simulink model "untitled1"  (R2024a)
settings: Solver=VariableStepAuto  StartTime=0.0  StopTime=10.0  RelTol=1e-3
undefined symbols (not defined in the file or in its folder): Discrete, pInitialization, Time
libraries: ctrlSharedLib x11, simulink x6
settings Model: Creator=DELL  LastModifiedBy=DELL

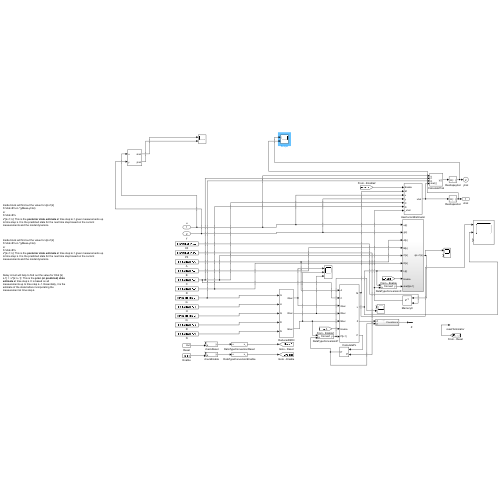
[thumbnail: Simulink's stored preview of the top-level diagram]
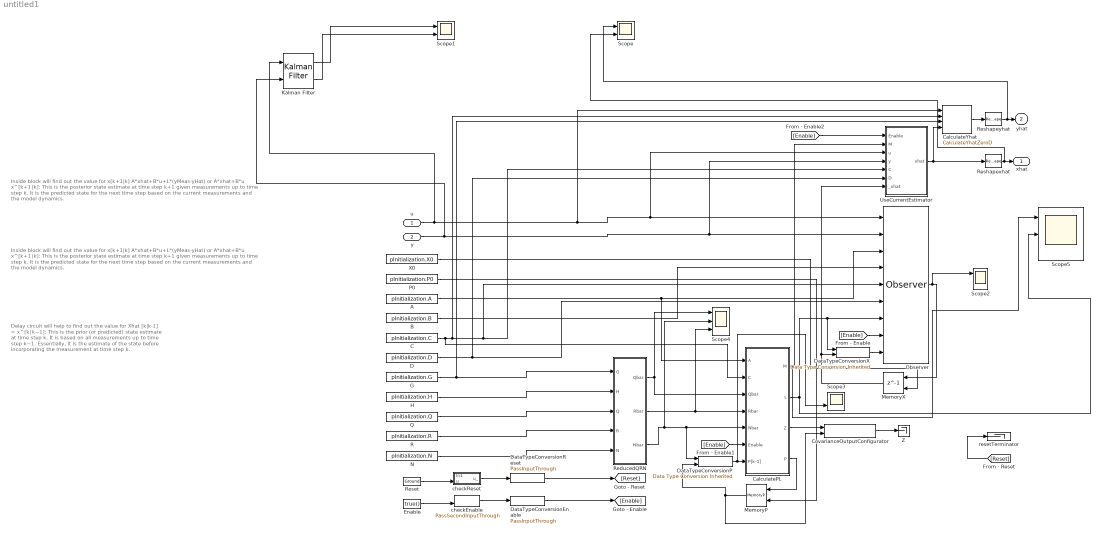
== system untitled1 ==
  note: Inside block will find out the value for x[k+1|k]
      | A*xhat+B*u+L*(yMeas-yHat)
      | or
      | A*xhat+B*u
      | x^[k+1∣k]: This is the posterior state estimate at time step k+1 given measurements up to time step k. It is the predicted state for the next time step based on the current measurements and the model dynamics.
  note: Inside block will find out the value for x[k+1|k]
      | A*xhat+B*u+L*(yMeas-yHat)
      | or
      | A*xhat+B*u
      | x^[k+1∣k]: This is the posterior state estimate at time step k+1 given measurements up to time step k. It is the predicted state for the next time step based on the current measurements and the model dynamics.
  note: Delay circuit will help to find out the value for Xhat [k|k-1] = x^[k∣k−1]: This is the prior (or predicted) state estimate at time step k. It is based on all measurements up to time step k−1. Essentially, it is the estimate of the state before incorporating the measurement at time step k.
  u : Inport
  y : Inport  Port=2
  A : Constant  Value=pInitialization.A  VectorParams1D=off  OutDataTypeStr=Inherit: Inherit via back propagation
  B : Constant  Value=pInitialization.B  VectorParams1D=off  OutDataTypeStr=Inherit: Inherit via back propagation
  C : Constant  Value=pInitialization.C  VectorParams1D=off  OutDataTypeStr=Inherit: Inherit via back propagation
  CalculatePL : Subsystem  mask(ctrlKalmanFilterConstantPL){}
      settings: LibrarySourceBlock=ctrlSharedLib/KalmanFilterUtilities/ConstantPL
  CalculateYhat : ctrlSharedLib/KalmanFilterUtilities/CalculateYhatZeroD  SystemSampleTime=-1  VariantActivationTime=update diagram  AllowFlexibleInterface=on  Latency=0  AutoFrameSizeCalculation=off
  CovarianceOutputConfigurator : ctrlSharedLib/Kalman Filter/CovarianceOutputConfigurator  SystemSampleTime=-1  VariantActivationTime=update diagram  AllowFlexibleInterface=on  Latency=0  AutoFrameSizeCalculation=off
  D : Constant  Value=pInitialization.D  VectorParams1D=off  OutDataTypeStr=Inherit: Inherit via back propagation
  DataTypeConversionEnable : ctrlSharedLib/Utilities/PassInputThrough  SystemSampleTime=-1  VariantActivationTime=update diagram  AllowFlexibleInterface=on  Latency=0  AutoFrameSizeCalculation=off
  DataTypeConversionP : simulink/Signal Attributes/Data Type Conversion Inherited  ConvertRealWorld=Real World Value  DoSatur=off
  DataTypeConversionReset : ctrlSharedLib/Utilities/PassInputThrough  SystemSampleTime=-1  VariantActivationTime=update diagram  AllowFlexibleInterface=on  Latency=0  AutoFrameSizeCalculation=off
  DataTypeConversionX : simulink/Signal Attributes/Data Type Conversion Inherited  ConvertRealWorld=Real World Value  DoSatur=off
  Enable : Constant  Value=true()  OutDataTypeStr=boolean
  G : Constant  Value=pInitialization.G  VectorParams1D=off  OutDataTypeStr=Inherit: Inherit via back propagation
  H : Constant  Value=pInitialization.H  VectorParams1D=off  OutDataTypeStr=Inherit: Inherit via back propagation
  Kalman Filter : ctrlSharedLib/Kalman Filter  TimeDomain=Discrete-Time  UseCurrentEstimator=off  ModelSource=Individual A, B, C, D matrices  ModelSourceVariable=ss(0.95,1,1,0,1)  A=[1.126900000000000,-0.494000000000000,0.112900000000000;1,0,0;0,1,0]  B=[-0.383200000000000;0.591900000000000;0.519100000000000]  C=[1,0,0]  D=0  NumberOfStates=1  NumberOfInputs=1  NumberOfOutputs=1  InitialEstimateSource=Dialog  X0=[1;0;0]  P0=10  UseK=off  UseGH=off  NumberOfProcessNoiseInputs=1  G=1  TimeInvariantG=on  H=0  TimeInvariantH=on  Q=2.300000000000000  TimeInvariantQ=on  R=10  TimeInvariantR=on  N=0  TimeInvariantN=on  AddInputPort=on  AddEnablePort=off  OutputEstimatedY=on  OutputP=off  Ts=-1
  MemoryP : ctrlSharedLib/KalmanFilterUtilities/MemoryP  SystemSampleTime=-1  VariantActivationTime=update diagram  AllowFlexibleInterface=on  Latency=0  AutoFrameSizeCalculation=off
  MemoryX : Delay  DelayLength=1  InitialConditionSource=Input port
      settings: InputPortMap=u0,p4
  N : Constant  Value=pInitialization.N  VectorParams1D=off  OutDataTypeStr=Inherit: Inherit via back propagation
  Observer : ctrlSharedLib/Kalman Filter/Observer  SystemSampleTime=-1  VariantActivationTime=update diagram  AllowFlexibleInterface=on  Latency=0  AutoFrameSizeCalculation=off
  P0 : Constant  Value=pInitialization.P0  OutDataTypeStr=Inherit: Inherit via back propagation
  Q : Constant  Value=pInitialization.Q  VectorParams1D=off  OutDataTypeStr=Inherit: Inherit via back propagation
  R : Constant  Value=pInitialization.R  VectorParams1D=off  OutDataTypeStr=Inherit: Inherit via back propagation
  ReducedQRN : Subsystem  mask(ctrlKalmanFilterNoReducedQRN){}
      settings: LibrarySourceBlock=ctrlSharedLib/KalmanFilterUtilities/NoReducedQRN
  Reset : ctrlSharedLib/Utilities/Ground  OutDataTypeStr=boolean  Dimensions=1
  Reshapexhat : Reshape
  Reshapeyhat : Reshape
  Scope{,1..3} (4 alike) : Scope  NumInputPorts=2
  Scope4 : Scope  NumInputPorts=3
  Scope5 : Scope  NumInputPorts=3
  UseCurrentEstimator : Subsystem  mask(ctrlKalmanFilterDontUseCurrentEstimator){}
      settings: LibrarySourceBlock=ctrlSharedLib/KalmanFilterUtilities/DontUseCurrentEstimator
  X0 : Constant  Value=pInitialization.X0  VectorParams1D=off  OutDataTypeStr=Inherit: Inherit via back propagation
  Z : Terminator
  checkEnable : ctrlSharedLib/KalmanFilterUtilities/PassSecondInputThrough  SystemSampleTime=-1  VariantActivationTime=update diagram  AllowFlexibleInterface=on  Latency=0  AutoFrameSizeCalculation=off
  checkReset : Subsystem  mask(ctrlKalmanFilterPassSecondInputThrough){}
      settings: LibrarySourceBlock=ctrlSharedLib/KalmanFilterUtilities/PassSecondInputThrough
      mask Display:
      | port_label('Input',2,'u');
      | port_label('Output',1,'y');
  resetTerminator : Terminator
  xhat : Outport  VectorParamsAs1DForOutWhenUnconnected=off
  yhat : Outport  Port=2
  wires:
  CalculatePL/1(M) -> Scope5/1, UseCurrentEstimator/2(M)
  P0/1 -> MemoryP/2
  Observer/1 -> Scope2/1, MemoryX/1
  DataTypeConversionReset/1 -> [Reset]
  [Enable] -> CalculatePL/6(Enable)
  DataTypeConversionEnable/1 -> [Enable]
  Enable/1 -> checkEnable/2
  Reset/1 -> checkReset/2(u)
  checkEnable/1 -> DataTypeConversionEnable/1
  [Enable] -> Observer/8
  DataTypeConversionX/1 -> Observer/9
  CalculatePL/4(P) -> MemoryP/1
  CalculateYhat/1 -> Reshapeyhat/1
  ReducedQRN/2(Rbar) -> Scope4/3, CalculatePL/4(Rbar)
  [Enable] -> UseCurrentEstimator/1(Enable)
  checkReset/1(u_) -> DataTypeConversionReset/1
  MemoryX/1 -> DataTypeConversionX/2, UseCurrentEstimator/7(_xhat)
  CovarianceOutputConfigurator/1 -> Z/1
  Reshapeyhat/1 -> Scope/1, yhat/1
  [Reset] -> resetTerminator/1
  CalculatePL/3(Z) -> CovarianceOutputConfigurator/1
  UseCurrentEstimator/1(xhat) -> Reshapexhat/1, CalculateYhat/4
  ReducedQRN/1(Qbar) -> Scope4/1, CalculatePL/3(Qbar)
  CalculatePL/2(L) -> Observer/7, DataTypeConversionX/1, Scope5/2
  X0/1 -> MemoryX/2
  y/1 -> Kalman Filter/2, UseCurrentEstimator/4(y), Observer/2
  C/1 -> CalculatePL/2(C), CalculateYhat/2, Observer/5, UseCurrentEstimator/5(C)
  D/1 -> Observer/6, UseCurrentEstimator/6(D)
  G/1 -> CalculateYhat/3, ReducedQRN/1(G)
  H/1 -> ReducedQRN/2(H)
  Q/1 -> ReducedQRN/3(Q)
  R/1 -> ReducedQRN/4(R)
  N/1 -> ReducedQRN/5(N)
  B/1 -> Observer/4
  A/1 -> CalculatePL/1(A), Observer/3
  u/1 -> Kalman Filter/1, CalculateYhat/1, UseCurrentEstimator/3(u), Observer/1
  Kalman Filter/1 -> Scope1/1
  Reshapexhat/1 -> Scope/2, xhat/1
  DataTypeConversionP/1 -> Scope3/2, CalculatePL/7(P[k-1])
  ReducedQRN/3(Nbar) -> Scope4/2, CalculatePL/5(Nbar), DataTypeConversionP/1
  MemoryP/1 -> DataTypeConversionP/2, CovarianceOutputConfigurator/2
  Kalman Filter/2 -> Scope1/2

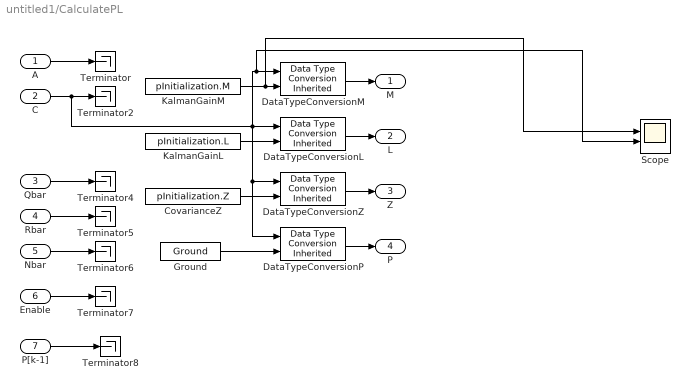
== system untitled1/CalculatePL ==
  A : Inport
  C : Inport  Port=2
  Qbar : Inport  Port=3
  Rbar : Inport  Port=4
  Nbar : Inport  Port=5
  Enable : Inport  Port=6
  P[k-1] : Inport  Port=7
  CovarianceZ : Constant  Value=pInitialization.Z
  DataTypeConversionL : simulink/Signal Attributes/Data Type Conversion Inherited  ConvertRealWorld=Real World Value  DoSatur=off
  DataTypeConversionM : simulink/Signal Attributes/Data Type Conversion Inherited  ConvertRealWorld=Real World Value  DoSatur=off
  DataTypeConversionP : simulink/Signal Attributes/Data Type Conversion Inherited  ConvertRealWorld=Real World Value  DoSatur=off
  DataTypeConversionZ : simulink/Signal Attributes/Data Type Conversion Inherited  ConvertRealWorld=Real World Value  DoSatur=off
  Ground : ctrlSharedLib/Utilities/Ground  OutDataTypeStr=single  Dimensions=1
  KalmanGainL : Constant  Value=pInitialization.L
  KalmanGainM : Constant  Value=pInitialization.M
  Scope : Scope  NumInputPorts=4
  Terminator{,2,4..8} (7 alike) : Terminator
  M : Outport  VectorParamsAs1DForOutWhenUnconnected=off
  L : Outport  Port=2  VectorParamsAs1DForOutWhenUnconnected=off
  Z : Outport  Port=3  VectorParamsAs1DForOutWhenUnconnected=off
  P : Outport  Port=4  VectorParamsAs1DForOutWhenUnconnected=off
  wires:
  DataTypeConversionP/1 -> P/1
  CovarianceZ/1 -> DataTypeConversionZ/2
  DataTypeConversionZ/1 -> Z/1
  Ground/1 -> DataTypeConversionP/2
  DataTypeConversionM/1 -> M/1
  KalmanGainM/1 -> Scope/2, DataTypeConversionM/2
  P[k-1]/1 -> Terminator8/1
  Enable/1 -> Terminator7/1
  KalmanGainL/1 -> DataTypeConversionL/2
  DataTypeConversionL/1 -> L/1
  Nbar/1 -> Terminator6/1
  Rbar/1 -> Terminator5/1
  Qbar/1 -> Terminator4/1
  C/1 -> Terminator2/1, DataTypeConversionL/1, Scope/3, DataTypeConversionM/1, DataTypeConversionZ/1, DataTypeConversionP/1
  A/1 -> Terminator/1

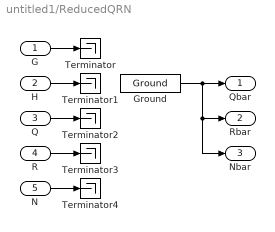
== system untitled1/ReducedQRN ==
  G : Inport  SampleTime=pInitialization.Ts
  H : Inport  Port=2  SampleTime=pInitialization.Ts
  Q : Inport  Port=3  SampleTime=pInitialization.Ts
  R : Inport  Port=4  SampleTime=pInitialization.Ts
  N : Inport  Port=5  SampleTime=pInitialization.Ts
  Ground : ctrlSharedLib/Utilities/Ground  OutDataTypeStr=single  Dimensions=1
  Terminator{,1..4} (5 alike) : Terminator
  Qbar : Outport  SampleTime=pInitialization.Ts  VectorParamsAs1DForOutWhenUnconnected=off
  Rbar : Outport  Port=2  SampleTime=pInitialization.Ts  VectorParamsAs1DForOutWhenUnconnected=off
  Nbar : Outport  Port=3  SampleTime=pInitialization.Ts  VectorParamsAs1DForOutWhenUnconnected=off
  wires:
  Ground/1 -> Rbar/1, Nbar/1, Qbar/1
  N/1 -> Terminator4/1
  R/1 -> Terminator3/1
  Q/1 -> Terminator2/1
  H/1 -> Terminator1/1
  G/1 -> Terminator/1

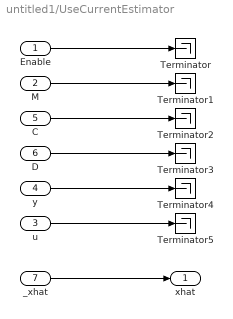
== system untitled1/UseCurrentEstimator ==
  Enable : Inport  SampleTime=pInitialization.Ts
  M : Inport  Port=2  SampleTime=pInitialization.Ts
  u : Inport  Port=3  SampleTime=pInitialization.Ts
  y : Inport  Port=4  SampleTime=pInitialization.Ts
  C : Inport  Port=5  SampleTime=pInitialization.Ts
  D : Inport  Port=6  SampleTime=pInitialization.Ts
  _xhat : Inport  Port=7  SampleTime=pInitialization.Ts
  Terminator{,1..5} (6 alike) : Terminator
  xhat : Outport  SampleTime=pInitialization.Ts  VectorParamsAs1DForOutWhenUnconnected=off
  wires:
  _xhat/1 -> xhat/1
  u/1 -> Terminator5/1
  y/1 -> Terminator4/1
  D/1 -> Terminator3/1
  C/1 -> Terminator2/1
  M/1 -> Terminator1/1
  Enable/1 -> Terminator/1

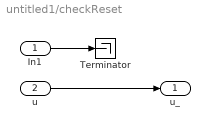
== system untitled1/checkReset ==
  In1 : Inport
  u : Inport  Port=2
  Terminator : Terminator
  u_ : Outport  VectorParamsAs1DForOutWhenUnconnected=off
  wires:
  In1/1 -> Terminator/1
  u/1 -> u_/1
